simulink model "macchina_asincrona_script_matlab_ok"  (R2023b)
settings: Solver=VariableStepAuto  StartTime=0.0  StopTime=10  RelTol=1e-3
libraries: simulink x2, spsAsynchronousMachineSIUnitsLib x1, spsSampleandHoldLib x1, spsThreePhaseSourceLib x1, sps_lib x1
settings Model: SnapshotInterval=2  Creator=simon  LastModifiedBy=simon
settings DataIOCC: ReturnWorkspaceOutputs=off

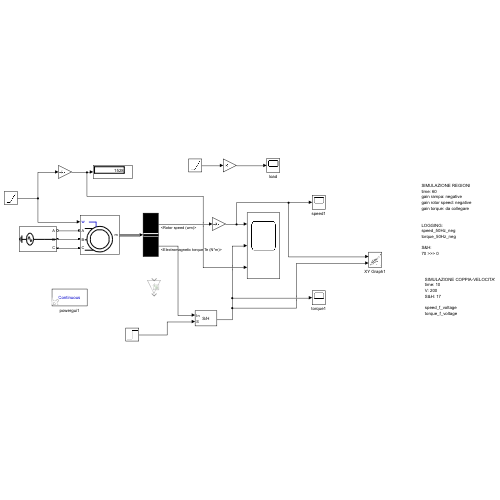
[thumbnail: Simulink's stored preview of the top-level diagram]
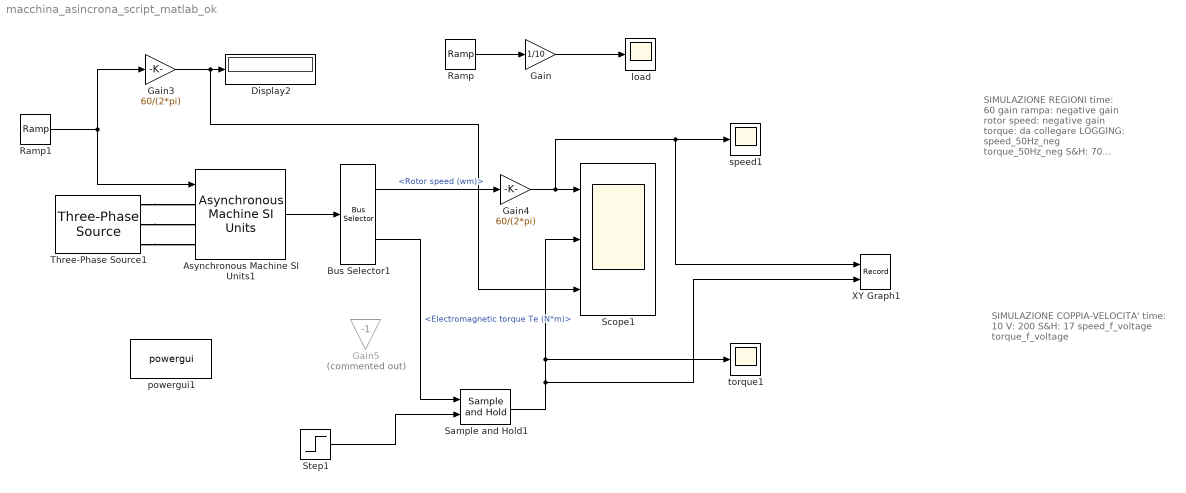
== system macchina_asincrona_script_matlab_ok ==
  note: SIMULAZIONE COPPIA-VELOCITA'
      | time: 10
      | V: 200
      | S&H: 17
      |
      | speed_f_voltage
      | torque_f_voltage
  note: SIMULAZIONE REGIONI
      | time: 60
      | gain rampa: negative
      | gain rotor speed: negative
      | gain torque: da collegare
      |
      |
      | LOGGING:
      | speed_50Hz_neg
      | torque_50Hz_neg
      |
      | S&H:
      | 70 >>> 0
  Asynchronous Machine SI Units1 : spsAsynchronousMachineSIUnitsLib/Asynchronous Machine SI Units  RotorType=Squirrel-cage  PresetModel="15:  5.4 HP (4KW)   400 V  50Hz 1430 RPM"  MechanicalLoad=Speed w  ShowDetailedParameters=on  ReferenceFrame=Stationary  Units=SI  MeasurementBus=off  NominalParameters=[4000 400 50]  VoltageRatio=1  Stator=[1.405 0.005839]  Rotor=[1.395 0.005839]  Cage1=[0.4155 0.002066]  Cage2=[0.4168 0.0003495]  Lm=0.1722  Mechanical=[0.0131 0.002985 2]  PolePairs=2  InitialConditions=[0 0 0 0 0 0 0 0]  SimulateSaturation=off  Saturation=[14.03593122, 27.81365428, 53.79336849, 72.68890987, 97.98006896, 148.6815601, 215.7428561, 302.9841135, 428.7778367 ; 230, 322, 414, 460, 506, 552, 598, 644, 690]  LoadFlowParameters=1492000  TsPowergui=0  TsBlock=-1  IterativeModel=Trapezoidal non iterative  IterativeDiscreteModel=Trapezoidal non iterative  Pmec=1.492e+006
  Bus Selector1 : BusSelector  OutputSignals=Mechanical.Rotor speed (wm),Mechanical.Electromagnetic torque Te (N*m)
  Display2 : Display
  Gain : Gain  Gain=1/10
  Gain3 : Gain  Gain=60/(2*pi)
  Gain4 : Gain  Gain=60/(2*pi)
  Gain5 : Gain  Commented=on  Gain=-1
  Ramp : simulink/Sources/Ramp  slope=(5.4*746)/(1430*pi/30)  start=0  InitialOutput=0
  Ramp1 : simulink/Sources/Ramp  slope=16  start=0  InitialOutput=0
  Sample and Hold1 : spsSampleandHoldLib/Sample and Hold  ic=70  Ts=0
      settings: LibrarySourceBlock=|
      | sps_lib/Control/Sample and
      | Hold
  Scope1 : Scope  NumInputPorts=3
  Step1 : Step  SampleTime=0
  Three-Phase Source1 : spsThreePhaseSourceLib/Three-Phase Source  InternalConnection=Yg  VoltagePhases=off  Voltage=400  PhaseAngle=0  Voltage_phases=[25e3 25e3 25e3]/sqrt(3)  PhaseAngles_phases=[0 -120 +120]  Frequency=50  NonIdealSource=off  SpecifyImpedance=off  Resistance=0.8929  Inductance=16.58e-3  ShortCircuitLevel=100e6  BaseVoltage=25e3  XRratio=7  BusType=swing  Pref=10e3  Qref=0  Prefabc=[10e3, 10e3, 10e3]  Qrefabc=[0, 0, 0]  Qmin=-inf  Qmax=inf
  XY Graph1 : Record  FileSettingsInternal="{\"entries\":[{\"content\":{\"excelSettings\":{\"content\":{},\"type\":\"Streamout.ExcelSettings\"}},\"type\":\"Streamout.FileSettingStorage\",\"uuid\":\"\"}],\"packageUris\":[\"http:\\/\\/schema.mathworks.com\\/mf0\\/streamout_blocks\\/R2020a\"],\"version\":\"1.0\"}"  Layout=[1 1]  SignalsInternal="{\"entries\":[{\"content\":{\"signals\":[{\"content\":{\"blockPath\":[],\"dimensions\":[1],\"domain\":\"\",\"lineColor\":\"#b746ff\",\"port\":1,\"sid\":[\"\"],\"signalID\":116,\"signalName\":\"Gain4\"},\"type\":\"RecordBlkView.Signal\",\"uuid\":\"\"},{\"content\":{\"blockPath\":[],\"dimensions\":[1],\"domain\":\"\",\"lineColor\":\"#64d413\",\"port\":2,\"sid\":[\"\"],\"signalID\":120,\"signalName\":\"Sample and\\nHold1\"},\"type\":\"RecordBlkView.Signal\",\"uuid\":\"\"}]},\"type\":\"RecordBlkView.InputSignals\",\"uuid\":\"\"}],\"packageUris\":[\"http:\\/\\/schema.mathworks.com\\/mf0\\/streamout_blocks\\/R2020a\"],\"version\":\"1.0\"}"  VisualizationBindings="{\"xyplotplugin\":{\"info\":[{\"series\":[],\"subplotID\":1}]}}"  CompatibilityTag=XY  st=-1
  load : Scope
  powergui1 : sps_lib/powergui  Priority=1  SimulationMode=Continuous  SampleTime=50e-6  frequency=60  Iterations=50  frequencyindice=50  Pbase=100e6  ErrMax=1e-4  UnitsV=kV  UnitsW=MW  buscounter=0  FunctionMessages=off  echomessages=off  EnableUseOfTLC=off  CurrentSourceSwitches=off  DisableSnubberDevices=off  DisableRonSwitches=off  DisableVfSwitches=off  DisplayEquations=off  AutomaticDiscreteSolvers=off  SolverType=Tustin/Backward Euler (TBE)  Interpol=off  ExternalGateDelay=off  methode=off  Ts=100  x0status=blocks  SPID=on  SwTol=0  HookPort=off  NonlinearTolerance=1e-4  nMaxIteration=100  ContinueOnMaxIteration=off  RestoreLinks=warning  ResistiveCurrentMeasurement=off  Frange=[0:2:500]  Ylog=off  Xlog=on  ShowGrid=off  save=off  variable=ZData  structure=0  ZoomFFT=off  StartTime=0.0  cycles=1  DisplayStyle=1  fundamental=60  FreqAxis=off  MaxFrequency=1000  frequencyindicesteady=1  RmsSteady=1  display=off
  speed1 : Scope
  torque1 : Scope
  wires:
  Asynchronous Machine SI Units1/1 -> Bus Selector1/1
  Ramp1/1 -> Asynchronous Machine SI Units1/1, Gain3/1
  Sample and Hold1/1 -> XY Graph1/2, Scope1/2, torque1/1
  Bus Selector1/2 -> Sample and Hold1/1  "<Electromagnetic torque Te (N*m)>"
  Step1/1 -> Sample and Hold1/2
  Bus Selector1/1 -> Gain4/1  "<Rotor speed (wm)>"
  Gain3/1 -> Scope1/3, Display2/1
  Gain4/1 -> XY Graph1/1, speed1/1, Scope1/1
  Gain/1 -> load/1
  Ramp/1 -> Gain/1
  connections:
  Three-Phase Source1/RConn2 -- Asynchronous Machine SI Units1/LConn2
  Three-Phase Source1/RConn1 -- Asynchronous Machine SI Units1/LConn1
  Three-Phase Source1/RConn3 -- Asynchronous Machine SI Units1/LConn3
